simulink model "ErikSchneider_prj_2_5_task2"  (R2025a)
settings: Solver=VariableStepAuto  StartTime=0.0  StopTime=10.0  RelTol=1e-3
libraries: slpidlib x1
settings Model: Creator=eriks  LastModifiedBy=eriks

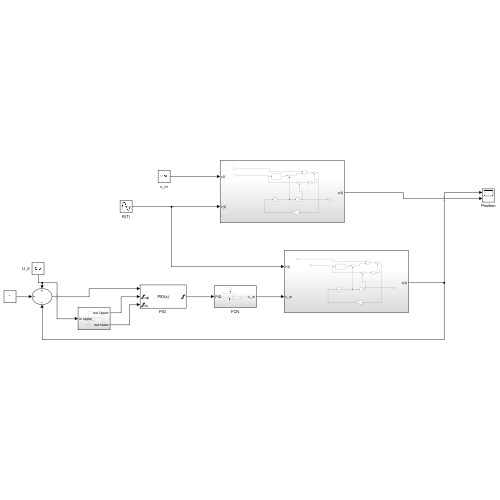
[thumbnail: Simulink's stored preview of the top-level diagram]
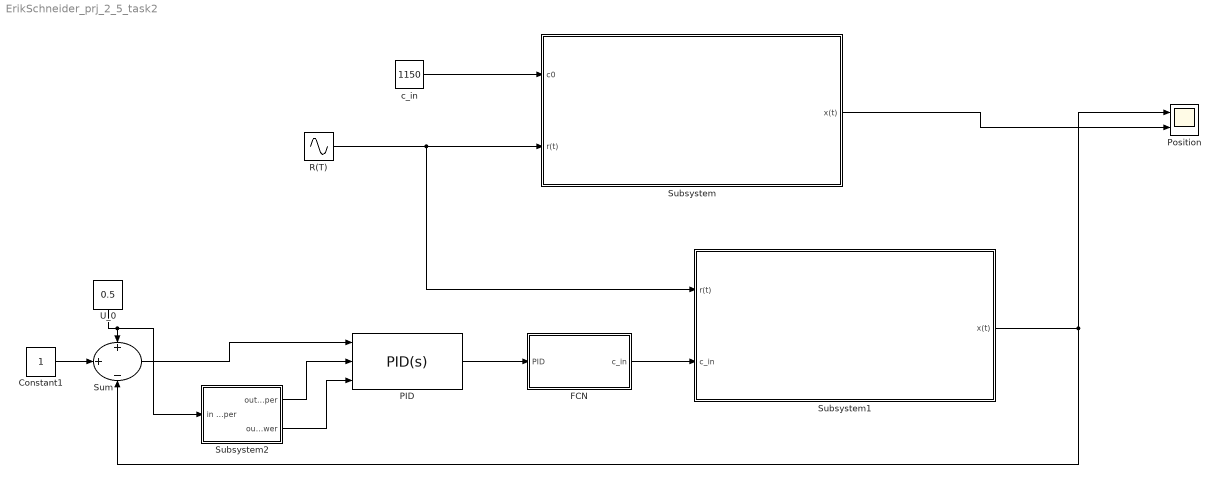
== system ErikSchneider_prj_2_5_task2 ==
  Constant1 : Constant
  FCN : Subsystem
  "PID " : slpidlib/PID Controller  Controller=PID  Form=Parallel  TimeDomain=Continuous-time  UseExternalTs=off  SampleTime=-1  IntegratorMethod=Forward Euler  FilterMethod=Forward Euler  ControllerParametersSource=internal  P=200  I=500  UseKiTs=off  D=1  UseExternalDerivativeSource=off  N=100  UseFilter=on  TunerSelectOption=Transfer Function Based (PID Tuner App)  InitialConditionSource=internal  InitialConditionForIntegrator=0  InitialConditionForFilter=0  DifferentiatorICPrevScaledInput=0  ExternalReset=none  TrackingMode=off  Kt=1  LimitOutput=on  SatLimitsSource=external  UpperSaturationLimit=inf  LowerSaturationLimit=-inf  LinearizeAsGain=on  AntiWindupMode=back-calculation  Kb=1  LimitIntegrator=on  UpperIntegratorSaturationLimit=inf  LowerIntegratorSaturationLimit=-inf  POutMin=[]  POutMax=[]  IOutMin=[]  IOutMax=[]  DOutMin=[]  DOutMax=[]  NOutMin=[]  NOutMax=[]  SumOutMin=[]  SumOutMax=[]  SaturationOutMin=[]  SaturationOutMax=[]  PParamMin=[]  PParamMax=[]  IParamMin=[]  IParamMax=[]  DParamMin=[]  DParamMax=[]  NParamMin=[]  NParamMax=[]  KbParamMin=[]  KbParamMax=[]  KtParamMin=[]  KtParamMax=[]  KbOutMin=[]  KbOutMax=[]  KtOutMin=[]  KtOutMax=[]  IntegratorOutMin=[]  IntegratorOutMax=[]  FilterOutMin=[]  FilterOutMax=[]  SumI1OutMin=[]  SumI1OutMax=[]  SumI2OutMin=[]  SumI2OutMax=[]  SumI3OutMin=[]  SumI3OutMax=[]  SumI4OutMin=[]  SumI4OutMax=[]  SumDOutMin=[]  SumDOutMax=[]  DifferentiatorOutMin=[]  DifferentiatorOutMax=[]  FilterDiffOutCoefMin=[]  FilterDiffOutCoefMax=[]  ReciprocalOutMin=[]  ReciprocalOutMax=[]  SumDenOutMin=[]  SumDenOutMax=[]  SumNumOutMin=[]  SumNumOutMax=[]  DivideOutMin=[]  DivideOutMax=[]  UdiffTsProdOutMin=[]  UdiffTsProdOutMax=[]  NTsProdOutMin=[]  NTsProdOutMax=[]  UintegralTsProdOutMin=[]  UintegralTsProdOutMax=[]  UngainTsProdOutMin=[]  UngainTsProdOutMax=[]  ClampingZeroOutDataTypeStr=Inherit: Inherit via back propagation  ClampingZeroOutMin=[]  ClampingZeroOutMax=[]  FilterDenConstantOutDataTypeStr=Inherit: Inherit via back propagation  FilterDenConstantOutMin=[]  FilterDenConstantOutMax=[]  PCopyOutDataTypeStr=Inherit: Inherit via back propagation  PCopyOutMin=[]  PCopyOutMax=[]  NCopyOutDataTypeStr=Inherit: Inherit via back propagation  NCopyOutMin=[]  NCopyOutMax=[]  IntegratorContinuousStateAttributes=''  IntegratorStateMustResolveToSignalObject=off  IntegratorRTWStateStorageClass=Auto  FilterContinuousStateAttributes=''  FilterStateMustResolveToSignalObject=off  FilterRTWStateStorageClass=Auto  ParallelPVariant=InternalParameters  IdealPVariant=Disabled  IVariant=InternalParameters  DVariant=InternalParameters  IntegratorVariant=Continuous  SatVariant=External  AWVariant=BackCalculation  PCopyVariant=Disabled  TRVariant=Disabled  FdbkBlocksVariant=Forward  IdealPFdbkVariant=Disabled  SatFdbkVariant=Disabled  DerivativeFilterVariant=ContFilter  NVariant=InternalParameters  NCopyVariant=Disabled  FilterICVariant=InternalICsFilter  IntegratorICVariant=InternalICs  ExternalResetVariant=Disabled  TRSumVariant=Passthrough  SumFdbkVariant=Disabled  SumVariant=Sum_PID  TsampFilterVariant=InternalTs  TsampNgainVariant=Passthrough  TsampIntegralVariant=Disabled_SignalSpec  ExternalSaturationOutDataTypeStr=Inherit: Same as second input  DerivativeSourceVariant=ErrorSignal  PreIntVariant=InternalPreInt
  Position : Scope  NumInputPorts=2
      settings: ActiveDisplayYMinimum=-0.030953128480816931  ActiveDisplayYMaximum=0.022303614314494562
  R(T) : Sin  Amplitude=0.01  Frequency=10  SampleTime=0
  Subsystem : Subsystem
  Subsystem1 : Subsystem
  Subsystem2 : Subsystem
  Sum : Sum  Inputs=+|+|-
  U_0 : Constant  Value=0.5
  c_in : Constant  Value=1150
  wires:
  c_in/1 -> Subsystem/1(c0)
  R(T)/1 -> Subsystem1/1(r(t)), Subsystem/2(r(t))
  Subsystem/1(x(t)) -> Position/2
  Subsystem1/1(x(t)) -> Position/1, Sum/3
  U_0/1 -> Subsystem2/1(in upper), Sum/1
  Sum/1 -> "PID "/1
  Subsystem2/1(out Upper) -> "PID "/2
  Subsystem2/2(out lower) -> "PID "/3
  "PID "/1 -> FCN/1(PID)
  Constant1/1 -> Sum/2
  FCN/1(c_in) -> Subsystem1/2(c_in)

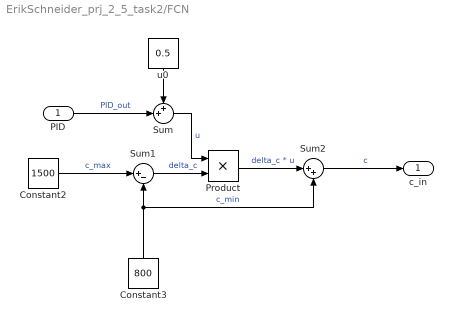
== system ErikSchneider_prj_2_5_task2/FCN ==
  PID : Inport
  Constant2 : Constant  Value=1500
  Constant3 : Constant  Value=800
  Product : Product
  Sum : Sum  Inputs=++|
  Sum1 : Sum  Inputs=|+-
  Sum2 : Sum  Inputs=|++
  u0 : Constant  Value=0.5
  c_in : Outport
  wires:
  Product/1 -> Sum2/1  "delta_c * u"
  Constant3/1 -> Sum2/2, Sum1/2  "c_min"
  Constant2/1 -> Sum1/1  "c_max"
  Sum2/1 -> c_in/1  "c"
  PID/1 -> Sum/2  "PID_out"
  Sum1/1 -> Product/2  "delta_c"
  u0/1 -> Sum/1
  Sum/1 -> Product/1  "u"

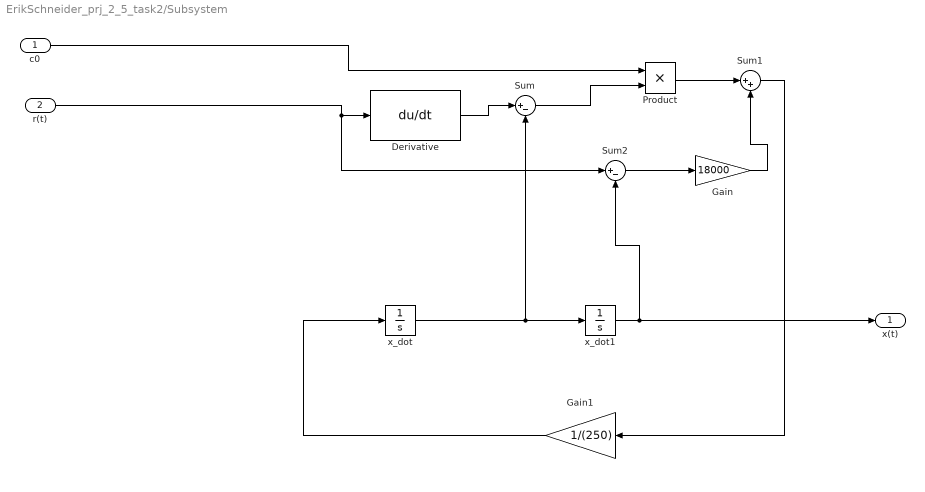
== system ErikSchneider_prj_2_5_task2/Subsystem ==
  c0 : Inport
  r(t) : Inport  Port=2
  Derivative : Derivative
  Gain : Gain  Gain=18000
  Gain1 : Gain  Gain=1/(250)
  Product : Product
  Sum : Sum  Inputs=|+-
  Sum1 : Sum  Inputs=|++
  Sum2 : Sum  Inputs=|+-
  x_dot : Integrator
  x_dot1 : Integrator
  x(t) : Outport
  wires:
  Sum2/1 -> Gain/1
  Derivative/1 -> Sum/1
  Product/1 -> Sum1/1
  Gain1/1 -> x_dot/1
  x_dot/1 -> Sum/2, x_dot1/1
  r(t)/1 -> Sum2/1, Derivative/1
  Sum/1 -> Product/2
  x_dot1/1 -> x(t)/1, Sum2/2
  Sum1/1 -> Gain1/1
  Gain/1 -> Sum1/2
  c0/1 -> Product/1

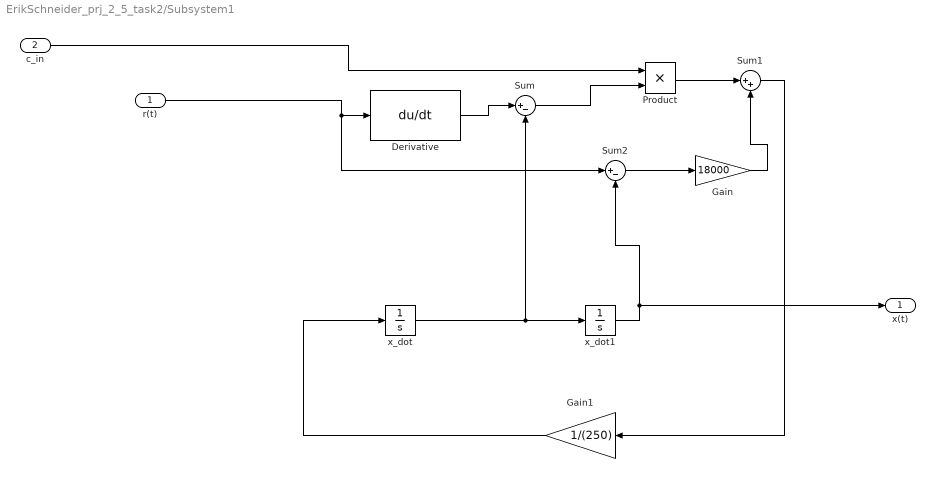
== system ErikSchneider_prj_2_5_task2/Subsystem1 ==
  r(t) : Inport
  c_in : Inport  Port=2
  Derivative : Derivative
  Gain : Gain  Gain=18000
  Gain1 : Gain  Gain=1/(250)
  Product : Product
  Sum : Sum  Inputs=|+-
  Sum1 : Sum  Inputs=|++
  Sum2 : Sum  Inputs=|+-
  x_dot : Integrator
  x_dot1 : Integrator
  x(t) : Outport
  wires:
  Sum2/1 -> Gain/1
  Derivative/1 -> Sum/1
  Product/1 -> Sum1/1
  Gain1/1 -> x_dot/1
  x_dot/1 -> Sum/2, x_dot1/1
  r(t)/1 -> Sum2/1, Derivative/1
  Sum/1 -> Product/2
  x_dot1/1 -> x(t)/1, Sum2/2
  Sum1/1 -> Gain1/1
  Gain/1 -> Sum1/2
  c_in/1 -> Product/1

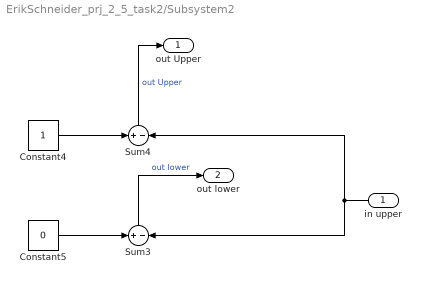
== system ErikSchneider_prj_2_5_task2/Subsystem2 ==
  in upper : Inport
  Constant4 : Constant
  Constant5 : Constant  Value=0
  Sum3 : Sum  Inputs=+|-
  Sum4 : Sum  Inputs=+-
  out Upper : Outport
  out lower : Outport  Port=2
  wires:
  Constant5/1 -> Sum3/1
  Constant4/1 -> Sum4/1
  in upper/1 -> Sum3/2, Sum4/2
  Sum4/1 -> out Upper/1  "out Upper"
  Sum3/1 -> out lower/1  "out lower"
